simulink model "MOT_CTRL_PTH_FUN_003_2"  (R2025a)
settings: Solver=VariableStepAuto  StartTime=0.0  StopTime=10.0  RelTol=1e-3
settings Model: DataDictionary=Hbridge.sldd  Creator=tecnicomcbti  LastModifiedBy=tecnicomcbti

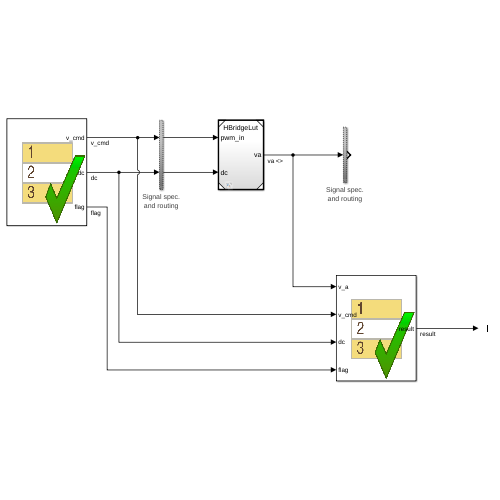
[thumbnail: Simulink's stored preview of the top-level diagram]
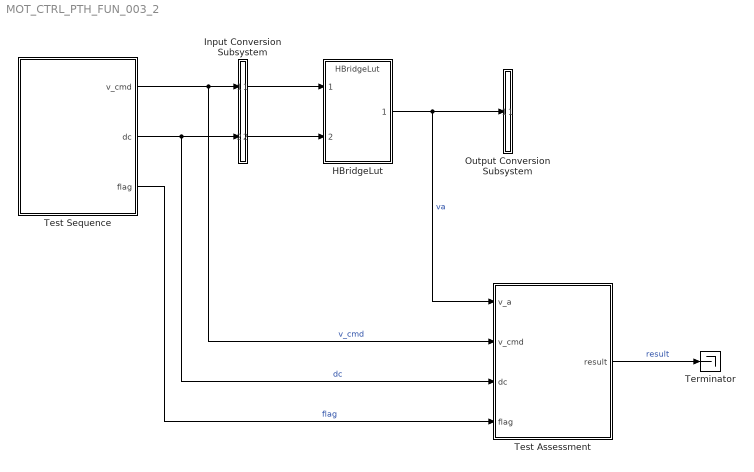
== system MOT_CTRL_PTH_FUN_003_2 ==
  HBridgeLut : ModelReference  ModelNameDialog=HBridgeLut  SimulationMode=Normal  ModelReferenceVersion=1.7
  Input Conversion Subsystem : Subsystem  Tag=__SLT_ICS__  Description=|
      | Signal spec.
      | and routing
      settings: AttributesFormatString=%<Description>
  Output Conversion Subsystem : Subsystem  Tag=__SLT_OCS__  Description=|
      | Signal spec.
      | and routing
      settings: AttributesFormatString=%<Description>
  Terminator : Terminator
  Test Assessment : Test Sequence  TreatAsAtomicUnit=on
  Test Sequence : Test Sequence  TreatAsAtomicUnit=on
  wires:
  Input Conversion Subsystem/1(Outport_1) -> HBridgeLut/1
  Input Conversion Subsystem/2(Outport_2) -> HBridgeLut/2
  HBridgeLut/1 -> Test Assessment/1(v_a), Output Conversion Subsystem/1(Inport_1)  "va"
  Test Assessment/1(result) -> Terminator/1  "result"
  Test Sequence/1(v_cmd) -> Test Assessment/2(v_cmd), Input Conversion Subsystem/1(Inport_1)  "v_cmd"
  Test Sequence/2(dc) -> Test Assessment/3(dc), Input Conversion Subsystem/2(Inport_2)  "dc"
  Test Sequence/3(flag) -> Test Assessment/4(flag)  "flag"

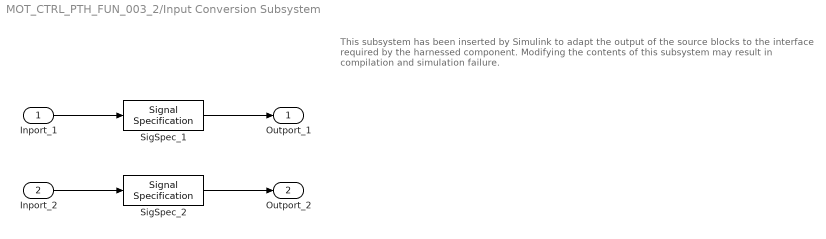
== system MOT_CTRL_PTH_FUN_003_2/Input Conversion Subsystem ==
  note: This subsystem has been inserted by Simulink to adapt the output of the source blocks to the interface required by the harnessed component.
      |  Modifying the contents of this subsystem may result in compilation and simulation failure.
  Inport_1 : Inport
  Inport_2 : Inport  Port=2
  SigSpec_1 : SignalSpecification  OutDataTypeStr=double  Dimensions=[1]  SampleTime=[0, 0]
  SigSpec_2 : SignalSpecification  OutDataTypeStr=double  Dimensions=[1]  SampleTime=[0, 0]
  Outport_1 : Outport
  Outport_2 : Outport  Port=2
  wires:
  SigSpec_1/1 -> Outport_1/1
  Inport_1/1 -> SigSpec_1/1
  SigSpec_2/1 -> Outport_2/1
  Inport_2/1 -> SigSpec_2/1

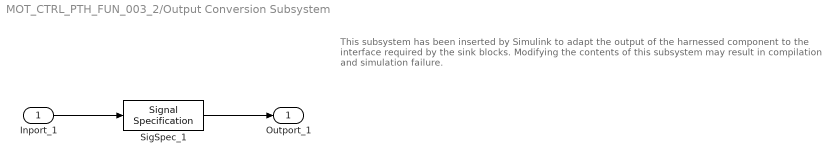
== system MOT_CTRL_PTH_FUN_003_2/Output Conversion Subsystem ==
  note: This subsystem has been inserted by Simulink to adapt the output of the harnessed component to the interface required by the sink blocks.
      |  Modifying the contents of this subsystem may result in compilation and simulation failure.
  Inport_1 : Inport
  SigSpec_1 : SignalSpecification  OutDataTypeStr=double  Dimensions=[1]
  Outport_1 : Outport
  wires:
  Inport_1/1 -> SigSpec_1/1
  SigSpec_1/1 -> Outport_1/1

== stateflow chart MOT_CTRL_PTH_FUN_003_2/Test Assessment ==
  state step_1
    state step_1_1
      if((dc==1) && (v_a < -v_max*0.95) && (v_a > -v_max*1.05))
      result=true;
      else
      result=false;
      end
    state step_1_2
    (default) -> (junction 22)
    step_1 -> (junction 22)
    (junction 22) -> (junction 23) [order 1] : [(flag && (v_cmd<0))
        | ]
    (junction 23) -> step_1_1 [order 1] : [~in(step_1.step_1_1)]
    (junction 22) -> (junction 31) [order 2]
    (junction 23) -> (junction 26) [order 2]
    (junction 31) -> (junction 32)
    (junction 32) -> step_1_2 [order 1] : [~in(step_1.step_1_2)]
    (junction 32) -> (junction 35) [order 2]
  (default) -> step_1
  data: v_a input; v_cmd input; dc input; flag input boolean; result output boolean; v_max constant double =336

== stateflow chart MOT_CTRL_PTH_FUN_003_2/Test Sequence ==
  state Start
    v_cmd=0;
    dc=0;
    flag=false;
  state Set_positive
    v_cmd=-5;
    dc=1;
    flag=true;
  (default) -> Start
  Start -> Set_positive : [
      | after(1,sec)
      | ]
  data: v_cmd output; dc output; flag output boolean
